simulink model "closed_observer"  (R2024a)
settings: Solver=VariableStepAuto  StartTime=0.0  StopTime=30  MaxStep=1e-4  RelTol=1e-4
values from neighbouring files (symbols this model uses):
  A = [5 -9 -7 1 ... (first row only)    [main3.m]
  B = [3 0 ... (first row only)    [main3.m]
  C = [2 -2 2 2 ... (first row only)    [main3.m]
  D = [0 4 ... (first row only)    [main3.m]
  L = PL * C' * inv(RL)    [main3.m]
  x0 = [1 1 1 1]'    [main3.m]
  x0_hat = [0 0 0 0]'    [main3.m]
undefined symbols (not defined in the file or in its folder): K
settings Model: Creator=eva  LastModifiedBy=eva

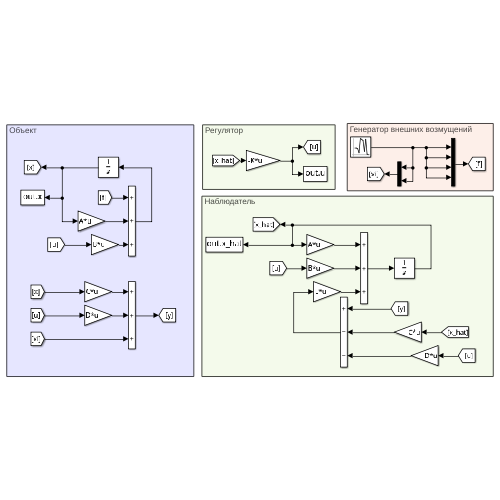
[thumbnail: Simulink's stored preview of the top-level diagram]
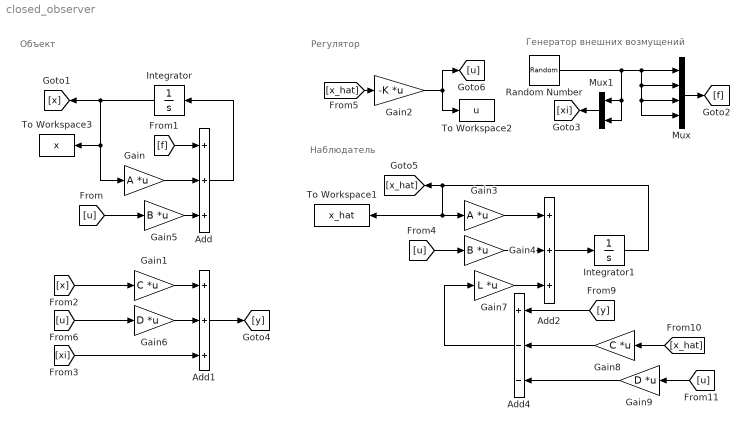
== system closed_observer ==
  note: Регулятор
  note: Объект
  note: Наблюдатель
  note: Генератор внешних возмущений
  Add : Sum  Inputs=+++
  Add1 : Sum  Inputs=+++
  Add2 : Sum  Inputs=+++
  Add4 : Sum  Inputs=+--
  Gain : Gain  Gain=A  Multiplication=Matrix(K*u)
  Gain1 : Gain  Gain=C  Multiplication=Matrix(K*u)
  Gain2 : Gain  Gain=-K  Multiplication=Matrix(K*u)
  Gain3 : Gain  Gain=A  Multiplication=Matrix(K*u)
  Gain4 : Gain  Gain=B  Multiplication=Matrix(K*u)
  Gain5 : Gain  Gain=B  Multiplication=Matrix(K*u)
  Gain6 : Gain  Gain=D  Multiplication=Matrix(K*u)
  Gain7 : Gain  Gain=L  Multiplication=Matrix(K*u)
  Gain8 : Gain  Gain=C  Multiplication=Matrix(K*u)
  Gain9 : Gain  Gain=D  Multiplication=Matrix(K*u)
  Integrator : Integrator  InitialCondition=x0
  Integrator1 : Integrator  InitialCondition=x0_hat
  Mux : Mux
  Mux1 : Mux  Inputs=2
  Random Number : RandomNumber  Variance=0.1  Seed=23341  SampleTime=0.01
  To Workspace1 : ToWorkspace  VariableName=x_hat  SaveFormat=Structure With Time  SampleTime=-1
  To Workspace2 : ToWorkspace  VariableName=u  SaveFormat=Structure With Time  SampleTime=-1
  To Workspace3 : ToWorkspace  VariableName=x  SaveFormat=Structure With Time  SampleTime=-1
  wires:
  Random Number/1 -> Mux1/2, Mux1/1, Mux/1, Mux/4, Mux/3, Mux/2
  Add1/1 -> [y]
  Gain1/1 -> Add1/1
  Add/1 -> Integrator/1
  Mux/1 -> [f]
  [f] -> Add/1
  [x] -> Gain1/1
  Gain/1 -> Add/2
  [x_hat] -> Gain2/1
  Gain2/1 -> [u], To Workspace2/1
  Gain5/1 -> Add/3
  [u] -> Gain5/1
  Integrator/1 -> [x], To Workspace3/1, Gain/1
  [xi] -> Add1/3
  Gain6/1 -> Add1/2
  [u] -> Gain6/1
  Mux1/1 -> [xi]
  [u] -> Gain4/1
  Gain3/1 -> Add2/1
  Gain4/1 -> Add2/2
  Gain7/1 -> Add2/3
  [y] -> Add4/1
  Gain8/1 -> Add4/2
  [x_hat] -> Gain8/1
  [u] -> Gain9/1
  Gain9/1 -> Add4/3
  Add4/1 -> Gain7/1
  Add2/1 -> Integrator1/1
  Integrator1/1 -> To Workspace1/1, Gain3/1, [x_hat]
